simulink model "MAtlab file"  (R2018a)
settings: Solver=VariableStepAuto  StartTime=0.0  StopTime=1  RelTol=1e-3
libraries: powerlib x1
settings Model: Creator=hp  LastModifiedBy=hp

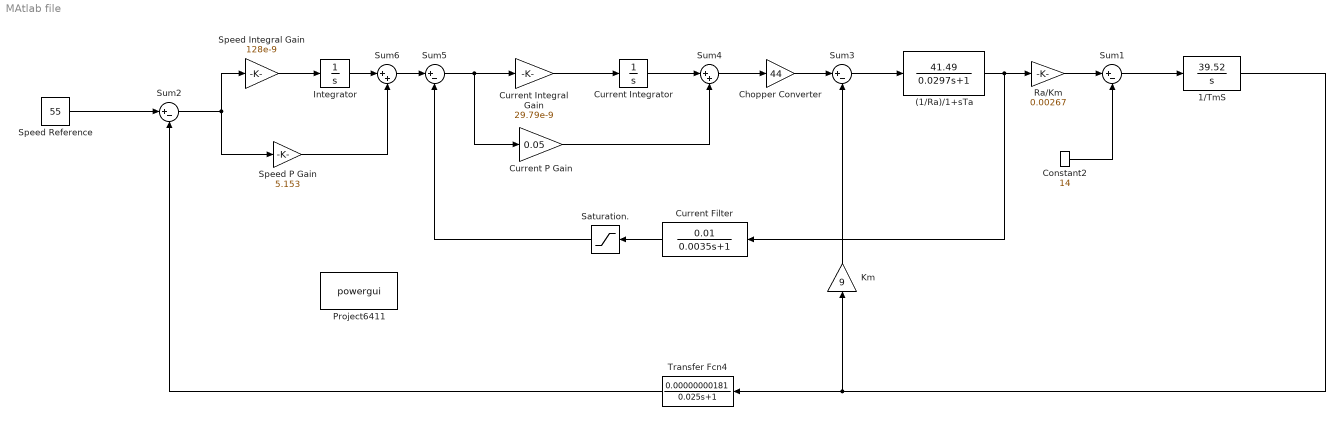
== system MAtlab file ==
  (1/Ra)/1+sTa : TransferFcn  Numerator=[41.49]  Denominator=[0.0297 1]
  1/TmS : TransferFcn  Numerator=[39.52]  Denominator=[1 0]
  Chopper Converter : Gain  Gain=44
  Constant2 : Constant  Value=14
  Current Filter : TransferFcn  Numerator=[0.01]  Denominator=[0.0035 1]
  Current Integral Gain : Gain  Gain=29.79e-9
  Current Integrator : Integrator
  Current P Gain : Gain  Gain=0.05
  "Integrator " : Integrator
  Km : Gain  Gain=9
  Project6411 : powerlib/powergui  Priority=1  SimulationMode=Continuous  SampleTime=50e-6  frequency=60  Iterations=50  frequencyindice=60  Pbase=100e6  ErrMax=1e-4  UnitsV=kV  UnitsW=MW  buscounter=0  FunctionMessages=off  echomessages=off  EnableUseOfTLC=off  CurrentSourceSwitches=off  DisableSnubberDevices=off  DisableRonSwitches=off  DisableVfSwitches=off  DisplayEquations=off  SolverType=Tustin/Backward Euler (TBE)  Interpol=off  ExternalGateDelay=off  methode=off  Ts=100  x0status=blocks  SPID=on  SwTol=0  HookPort=off  RestoreLinks=warning  ResistiveCurrentMeasurement=off  Frange=[0:2:500]  Ylog=off  Xlog=on  ShowGrid=off  save=off  variable=ZData  structure=0  ZoomFFT=off  StartTime=0.0  cycles=1  DisplayStyle=1  fundamental=60  FreqAxis=off  MaxFrequency=1000  frequencyindicesteady=1  RmsSteady=1  display=off
  Ra/Km : Gain  Gain=0.00267
  Saturation. : Saturate  UpperLimit=1  LowerLimit=0
  Speed Integral Gain : Gain  Gain=128e-9
  Speed P Gain : Gain  Gain=5.153
  Speed Reference : Constant  Value=55
  Sum{1..3,5} (4 alike) : Sum  Inputs=|+-
  Sum4 : Sum  Inputs=|++
  Sum6 : Sum  Inputs=|++
  Transfer Fcn4 : TransferFcn  Numerator=[0.00000000181]  Denominator=[0.025 1]
  wires:
  Sum1/1 -> 1/TmS/1
  Chopper Converter/1 -> Sum3/1
  Sum4/1 -> Chopper Converter/1
  Current Integrator/1 -> Sum4/1
  Current Integral Gain/1 -> Current Integrator/1
  Current P Gain/1 -> Sum4/2
  Sum5/1 -> Current P Gain/1, Current Integral Gain/1
  Current Filter/1 -> Saturation./1
  Saturation./1 -> Sum5/2
  Sum6/1 -> Sum5/1
  "Integrator "/1 -> Sum6/1
  Speed Integral Gain/1 -> "Integrator "/1
  Speed P Gain/1 -> Sum6/2
  Sum2/1 -> Speed P Gain/1, Speed Integral Gain/1
  Transfer Fcn4/1 -> Sum2/2
  1/TmS/1 -> Km/1, Transfer Fcn4/1
  Km/1 -> Sum3/2
  Speed Reference/1 -> Sum2/1
  (1/Ra)/1+sTa/1 -> Current Filter/1, Ra/Km/1
  Ra/Km/1 -> Sum1/1
  Sum3/1 -> (1/Ra)/1+sTa/1
  Constant2/1 -> Sum1/2
